simulink model "tutorial11_observer"  (R2025a)
settings: Solver=VariableStepAuto  StartTime=0.0  StopTime=5  RelTol=1e-3
settings Model: Creator=xing2  LastModifiedBy=xing2

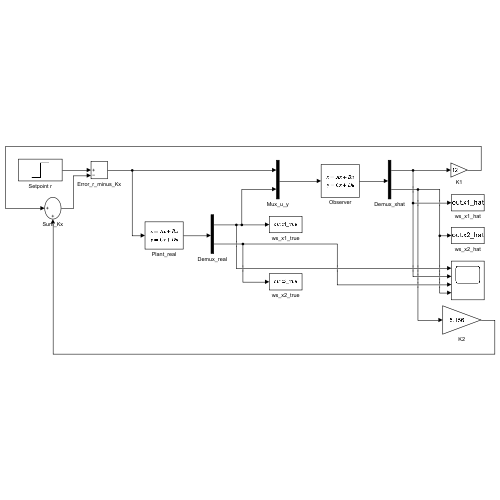
[thumbnail: Simulink's stored preview of the top-level diagram]
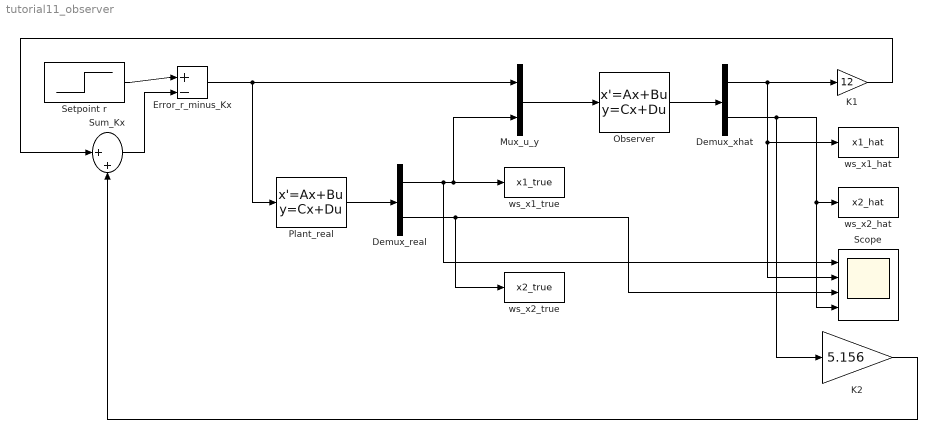
== system tutorial11_observer ==
  Demux_real : Demux  Outputs=2
  Demux_xhat : Demux  Outputs=2
  Error_r_minus_Kx : Sum  Inputs=|+-
  K1 : Gain  Gain=12
  K2 : Gain  Gain=5.156
  Mux_u_y : Mux  Inputs=2
  Observer : StateSpace  A=[-13.5 1;-41.2499999999999 -0.5]  B=[0 13.5;1 37.2499999999999]  C=[1 0;0 1]  D=[0 0;0 0]  InitialCondition=[0; 0]
  Plant_real : StateSpace  A=[0 1;-4 -0.5]  B=[0;1]  C=eye(2)  D=zeros(2,1)  InitialCondition=[0.3; 0]
  Scope : Scope  NumInputPorts=4
  Setpoint r : Step  Time=0.5  SampleTime=0
  Sum_Kx : Sum  Inputs=|++
  ws_x1_hat : ToWorkspace  VariableName=x1_hat  SaveFormat=Timeseries  SampleTime=-1
  ws_x1_true : ToWorkspace  VariableName=x1_true  SaveFormat=Timeseries  SampleTime=-1
  ws_x2_hat : ToWorkspace  VariableName=x2_hat  SaveFormat=Timeseries  SampleTime=-1
  ws_x2_true : ToWorkspace  VariableName=x2_true  SaveFormat=Timeseries  SampleTime=-1
  wires:
  Setpoint r/1 -> Error_r_minus_Kx/1
  Observer/1 -> Demux_xhat/1
  Sum_Kx/1 -> Error_r_minus_Kx/2
  Demux_real/1 -> Mux_u_y/2, ws_x1_true/1, Scope/1
  Plant_real/1 -> Demux_real/1
  Error_r_minus_Kx/1 -> Plant_real/1, Mux_u_y/1
  Demux_xhat/1 -> Scope/2, ws_x1_hat/1, K1/1
  Demux_real/2 -> Scope/3, ws_x2_true/1
  Mux_u_y/1 -> Observer/1
  Demux_xhat/2 -> Scope/4, ws_x2_hat/1, K2/1
  K1/1 -> Sum_Kx/1
  K2/1 -> Sum_Kx/2
